simulink model "Coefficients_Tuning"  (R2024a)
settings: Solver=VariableStepAuto  StartTime=0.0  StopTime=10.0  RelTol=1e-3
libraries: cstblocks x2
settings Model: Creator=gerar  LastModifiedBy=gerar

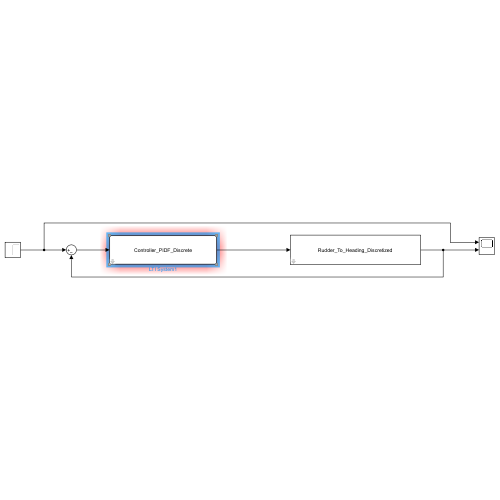
[thumbnail: Simulink's stored preview of the top-level diagram]
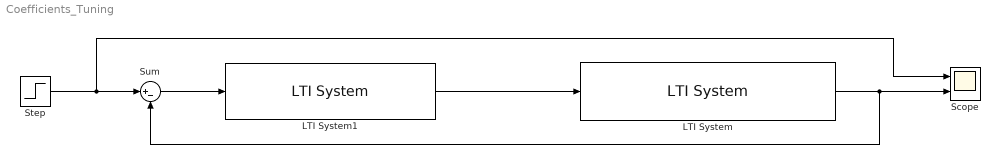
== system Coefficients_Tuning ==
  LTI System : cstblocks/LTI System  sys=Rudder_To_Heading_Discretized  IC=[]  PadeOrder=0
  LTI System1 : cstblocks/LTI System  sys=Controller_PIDF_Discrete  IC=[]  PadeOrder=0
  Scope : Scope  NumInputPorts=2
  Step : Step  After=15*(pi/180)  SampleTime=0
  Sum : Sum  Inputs=|+-
  wires:
  LTI System/1 -> Sum/2, Scope/2
  LTI System1/1 -> LTI System/1
  Sum/1 -> LTI System1/1
  Step/1 -> Scope/1, Sum/1
